simulink model "DCM_Test"  (R2019b)
settings: Solver=VariableStepAuto  StartTime=0.0  StopTime=0.03167  RelTol=1e-3
undefined symbols (not defined in the file or in its folder): D1, lagging, pulse
libraries: powerlib x12, powerlib_meascontrol x2, electricdrivelib x1
settings Model: Creator=Sy2  LastModifiedBy=Sy2
settings SolverCC: ZeroCrossAlgorithm=Adaptive
settings DebuggingCC: IgnoredZcDiagnostic=none

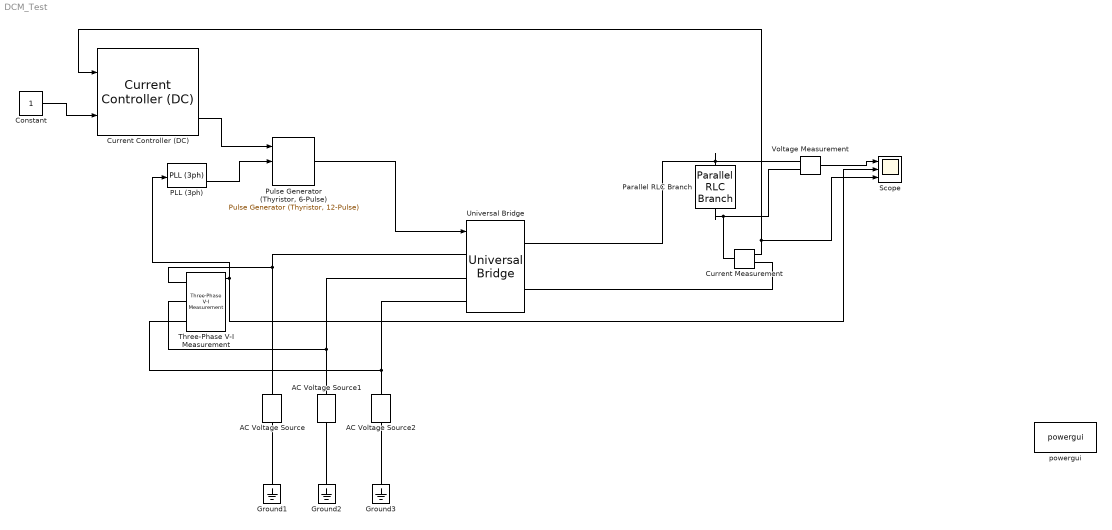
== system DCM_Test ==
  AC Voltage Source : powerlib/Electrical Sources/AC Voltage Source  Amplitude=480  Phase=0  Frequency=60  SampleTime=0  Measurements=None  BusType=swing  Pref=10e3  Qref=0  Qmin=-inf  Qmax=+inf
      settings: SourceProductName=Simscape Electrical
  AC Voltage Source1 : powerlib/Electrical Sources/AC Voltage Source  Amplitude=480  Phase=-120  Frequency=60  SampleTime=0  Measurements=None  BusType=swing  Pref=10e3  Qref=0  Qmin=-inf  Qmax=+inf
      settings: SourceProductName=Simscape Electrical
  AC Voltage Source2 : powerlib/Electrical Sources/AC Voltage Source  Amplitude=480  Phase=120  Frequency=60  SampleTime=0  Measurements=None  BusType=swing  Pref=10e3  Qref=0  Qmin=-inf  Qmax=+inf
      settings: SourceProductName=Simscape Electrical
  Constant : Constant
  Current Controller (DC) : electricdrivelib/Fundamental Drive Blocks/Current Controller (DC)  driveType=Rectifier based  detailLevel=Detailed  numQuadChop=2  numQuadRect=2  Pb=5*746  Vb=240  Kp=2  Ki=200  fci=500  F=5e3  lim=[20, 160]  sampling=20e-6  Ts=1e-6
      settings: SourceProductName=Simscape Electrical  SourceProductBaseCode=PS
  Current Measurement : powerlib/Measurements/Current Measurement  PhasorSimulation=off  OutputType=Complex  PSBequivalent=0
      settings: SourceProductName=Simscape Electrical
  Ground1 : powerlib/Elements/Ground  LConnTagsString=a
      settings: SourceProductName=Simscape Electrical
  Ground2 : powerlib/Elements/Ground  LConnTagsString=a
      settings: SourceProductName=Simscape Electrical
  Ground3 : powerlib/Elements/Ground  LConnTagsString=a
      settings: SourceProductName=Simscape Electrical
  PLL (3ph) : powerlib_meascontrol/PLL/PLL (3ph)  Fmin=45  Par_Init=[0, 60]  ParK=[180, 3200, 1]  TcD=1e-4  MaxRateChangeFreq=12  FilterCutOffFreq=25  Ts=0  AGC=on
      settings: SourceProductName=Simscape Electrical
  Parallel RLC Branch : powerlib/Elements/Parallel RLC Branch  LConnTagsString=a  RConnTagsString=__new0  BranchType=L  Resistance=30  Inductance=0.001  SetiL0=off  InitialCurrent=0  Capacitance=1e-6  Setx0=off  InitialVoltage=0  Measurements=None
      settings: SourceProductName=Simscape Electrical
  "Pulse Generator (Thyristor, 6-Pulse)" : powerlib_meascontrol/Pulse & Signal Generators/Pulse Generator (Thyristor, 12-Pulse)  GenType=6-pulse  Delta=D1 (lagging)  pwidth=60  Double_Pulse=off  Ts=0
      settings: SourceProductName=Simscape Electrical  SourceProductBaseCode=PS
  Scope : Scope  NumInputPorts=3
  Three-Phase V-I Measurement : powerlib/Measurements/Three-Phase V-I Measurement  VoltageMeasurement=phase-to-ground  SetLabelV=off  LabelV=Vabc  Vpu=off  VpuLL=off  CurrentMeasurement=yes  SetLabelI=off  LabelI=Iabc  Ipu=off  Pbase=100e6  Vbase=500e3  OutputType=Complex  PhasorSimulation=off  PSBequivalent=0
      settings: SourceProductName=Simscape Electrical
  Universal Bridge : powerlib/Power Electronics/Universal Bridge  Arms=3  SnubberResistance=1e5  SnubberCapacitance=inf  Device=Thyristors  Ron=1e-3  Lon=0  ForwardVoltages="[  0  0  ]"  ForwardVoltage=0  GTOparameters=[ 10e-6 , 20e-6 ]  IGBTparameters=[ 1e-6 , 2e-6 ]  Measurements=None  Measurements_2=None  converterType=Rectifier
      settings: SourceProductName=Simscape Electrical
  Voltage Measurement : powerlib/Measurements/Voltage Measurement  PhasorSimulation=off  OutputType=Complex  PSBequivalent=0
      settings: SourceProductName=Simscape Electrical
  powergui : powerlib/powergui  Priority=1  SimulationMode=Continuous  SampleTime=50e-6  frequency=60  Iterations=50  frequencyindice=60  Pbase=100e6  ErrMax=1e-4  UnitsV=kV  UnitsW=MW  buscounter=0  FunctionMessages=off  echomessages=off  EnableUseOfTLC=off  CurrentSourceSwitches=off  DisableSnubberDevices=off  DisableRonSwitches=off  DisableVfSwitches=off  DisplayEquations=off  AutomaticDiscreteSolvers=off  SolverType=Tustin/Backward Euler (TBE)  Interpol=off  ExternalGateDelay=off  methode=off  Ts=100  x0status=blocks  SPID=on  SwTol=0  HookPort=off  NonlinearTolerance=1e-4  nMaxIteration=100  ContinueOnMaxIteration=off  RestoreLinks=warning  ResistiveCurrentMeasurement=off  Frange=[0:2:500]  Ylog=off  Xlog=on  ShowGrid=off  save=off  variable=ZData  structure=0  ZoomFFT=off  StartTime=0.0  cycles=1  DisplayStyle=1  fundamental=60  FreqAxis=off  MaxFrequency=1000  frequencyindicesteady=1  RmsSteady=1  display=off
      settings: SourceProductName=Simscape Electrical
  wires:
  Voltage Measurement/1 -> Scope/1
  "Pulse Generator (Thyristor, 6-Pulse)"/1 -> Universal Bridge/1
  Three-Phase V-I Measurement/1 -> PLL (3ph)/1, Scope/2
  PLL (3ph)/2 -> "Pulse Generator (Thyristor, 6-Pulse)"/2
  Current Controller (DC)/3 -> "Pulse Generator (Thyristor, 6-Pulse)"/1
  Current Measurement/1 -> Scope/3, Current Controller (DC)/1
  Constant/1 -> Current Controller (DC)/2
  connections:
  Ground1/LConn1 -- AC Voltage Source/LConn1
  Ground2/LConn1 -- AC Voltage Source1/LConn1
  Ground3/LConn1 -- AC Voltage Source2/LConn1
  Parallel RLC Branch/LConn1 -- Universal Bridge/RConn1 -- Voltage Measurement/LConn1
  Parallel RLC Branch/RConn1 -- Current Measurement/LConn1 -- Voltage Measurement/LConn2
  AC Voltage Source2/RConn1 -- Universal Bridge/LConn3 -- Three-Phase V-I Measurement/LConn3
  AC Voltage Source1/RConn1 -- Universal Bridge/LConn2 -- Three-Phase V-I Measurement/LConn2
  AC Voltage Source/RConn1 -- Three-Phase V-I Measurement/LConn1 -- Universal Bridge/LConn1
  Current Measurement/RConn1 -- Universal Bridge/RConn2
